simulink model "Horno"  (R2015a)
settings: Solver=ode45  StartTime=0.0  StopTime=500.0  RelTol=1e-3
settings Model: Creator=Abel  LastModifiedBy=Abel

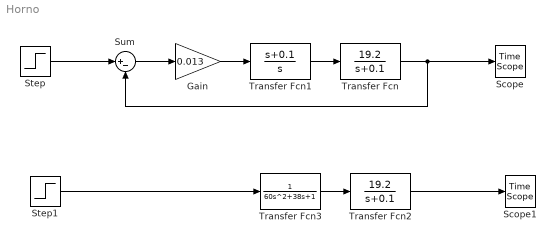
== system Horno ==
  Gain : Gain  Gain=0.013
  Scope : TimeScope
  Scope1 : TimeScope
  Step : Step  Time=0  SampleTime=0
  Step1 : Step  Time=0  SampleTime=0
  Sum : Sum  Inputs=|+-
  Transfer Fcn : TransferFcn  Numerator=[19.2]  Denominator=[1 0.1]
  Transfer Fcn1 : TransferFcn  Numerator=[1 0.1]  Denominator=[1 0]
  Transfer Fcn2 : TransferFcn  Numerator=[19.2]  Denominator=[1 0.1]
  Transfer Fcn3 : TransferFcn  Denominator=[60 38 1]
  wires:
  Sum/1 -> Gain/1
  Transfer Fcn/1 -> Sum/2, Scope/1
  Step/1 -> Sum/1
  Gain/1 -> Transfer Fcn1/1
  Transfer Fcn1/1 -> Transfer Fcn/1
  Transfer Fcn2/1 -> Scope1/1
  Transfer Fcn3/1 -> Transfer Fcn2/1
  Step1/1 -> Transfer Fcn3/1
